simulink model "Hexa_CAD_quaternion_ANSFT"  (R2024b)
settings: Solver=ode4  StartTime=0.0  StopTime=60  FixedStep=0.01  RelTol=1e-3
model workspace (MAT data in the model file):
  hover_2m = [0 0 2 0 0 0 0 0 2 0 0 0 ... (36 elements, 6x6)]
  square = [0 0 2.5 0 0 0 0 0 2.5 0 0 0 ... (36 elements, 6x6)]
  tf : Simulink.Parameter (value not decoded)
  tray0 = [0 0 0 0 0 0 0.2 0.15 2 0 0 0 ... (36 elements, 6x6)]
  tray1 = [0 0 0 0 0 0 0 0 2 0 0 0 ... (36 elements, 6x6)]
  tray2 = [0 0 0 0 0 0 2 0 5 0 0 0 ... (36 elements, 6x6)]
  tray3 = [0 0 0 0 0 0 2 0 5 0 0 0 ... (36 elements, 6x6)]
  tray4 = [0 0 0 0 0 0 2 0 5 0.15 0 0 ... (36 elements, 6x6)]
  tray5 = [0 0 0 0 0 0 0 0 5 0.15 0 0 ... (36 elements, 6x6)]
  tray_yaw = [0 0 0 0 0 0 0 0 5 0 0 0 ... (36 elements, 6x6)]
undefined symbols (not defined in the file or in its folder): F, Light, MIL, smiData, X, Y, Z
libraries: sm_lib x167, nesl_utility x29, dspobslib x9, sharedtransform x4, simulink x4, aerolibutil x3, matrix_library x1, sharedutil x1, robotcorelib x1, aerolibwind2 x1
(part 3 of 6)

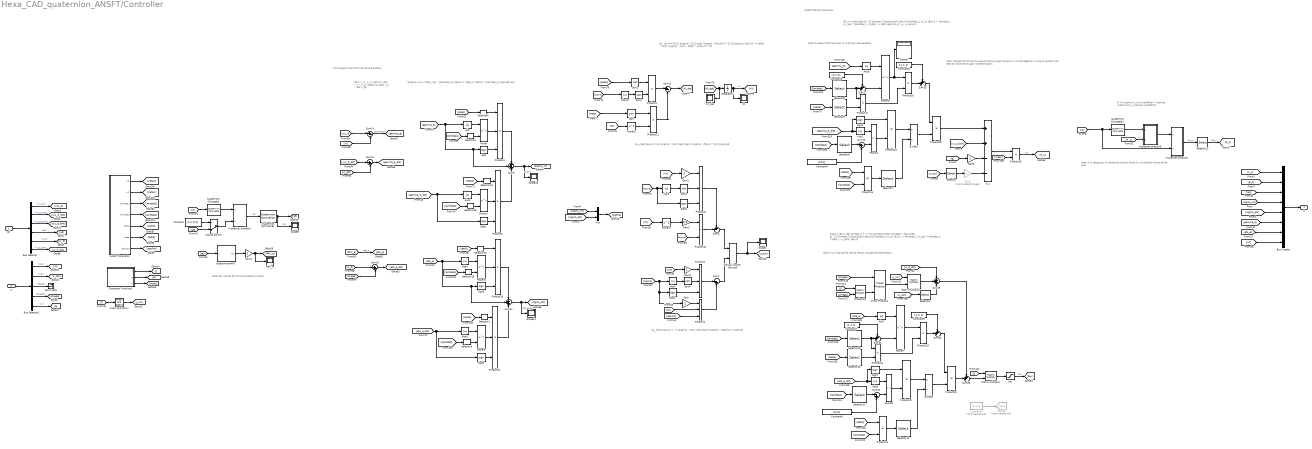
== system Hexa_CAD_quaternion_ANSFT/Controller ==
  note: $u_{\text{aux}}=-2K |\sigma|^{1/2} \text{sign} (\sigma) - \frac{K^2}{2}\sigma$
  note: $u_{\text{aux}} = - K |\sigma| ^{1/2} \text{sign}(\sigma) - 2\epsilon K \sigma$
  note: Note: PRV stands for Principal Rotation
      | Vector.
  note: $e = x_d - x_1 \\ \dot e = \dot x_d - x_2 \\ \ddot e = \ddot x_d - \dot x_2$
  note: Non-Singular Fast Terminal Sliding Surface
  note: $\sigma = e + \zeta_1 |e| ^{\lambda_1} sign(e) + \zeta_2 | \dot e| ^{\lambda_2} sign(\dot e)$
  note: $F_u = \frac{|\dot e|^{2-\lambda_2}\text{sign}(\dot e)}{\lambda_2 \xi_2} \Big (1 + \lambda_1 \xi_1|e|^{\lambda_1 - 1}\Big ) + \ddot \gamma_d - g - u_{aux}$
  note: Note: It seems that the mass is missing in
      | the equation.
  note: $\tau = \Big [ \dot \omega_d + J^{-1} \omega \times J \omega + \frac{|\dot e|^{2-\lambda_2}\text{sign}(\dot e)}{\lambda_2 \xi_2} \Big (1 + \lambda_1 \xi_1|e|^{\lambda_1 - 1}\Big ) - u_{aux} \Big ]$
  note: Note: Change the Thrust to a positive force, ergo the gravity will be negative,
      | will be using ENU over NED for future Simscape implementation.
  note: $^B \mathrm F_u = \mathbf{q}^*\otimes \mathrm{F}_u \otimes \mathbf q$
  note: ANSFT Position Controller
  note: Note: It is missing the Inertia Tensor outside
      | the parenthesis
  note: Note: It is necessary to rotate the control Force F_u
      | to the body frame of the FAH.
  note: $u_{aux}=-2K(t) |\sigma|^{1/2} sign (\sigma) - \frac{K(t)^2}{2}\sigma \\ \dot K(t) = \alpha ^{1/2} |\sigma| ^{1/2} - \beta ^{1/2}K(t)^2$
  qd : Inport
  q : Inport  Port=2
  ANSFT Constants : MATLAB Function  TreatAsAtomicUnit=on
  Abs{,1..10} (11 alike) : Abs  SaturateOnIntegerOverflow=off
  Bus Creator : BusCreator  Inputs=8
  Bus Selector : BusSelector  OutputSignals=xyz_d,xyz_d_dot,xyz_d_ddot,qd,w_d,w_d_dot
  Bus Selector1 : BusSelector  OutputSignals=pos,vel,bf_att,bf_datt,q
  Constant : Constant  Value=[1; 0; 0; 0]
  Constant{3,5,7,9} (4 alike) : Constant  Value=[1; 1; 1]
  Constant4 : Constant  Value=[2;2;2]
  Constant6 : Constant  Commented=on  Value=[0; 0; 0]
  Constant8 : Constant  Value=[2;2;2]
  Constants Functions : MATLAB Function  TreatAsAtomicUnit=on
  Cross Product1 : matrix_library/Cross Product
  Display : Display
  Divide2 : Product  Inputs=*/
  Divide3 : Product  Inputs=*/
  F_u : Sum  Inputs=++--
  Gain{,1,3..4} (4 alike) : Gain  Gain=2
  Gain2 : Gain  Gain=1/2
  Gain5 : Gain
  Gain6 : Gain  Commented=through  Gain=-1
  Goto59 : Goto  Commented=on  GotoTag=tau
  Integrator4 : Integrator  InitialCondition=[0;0;0; 0; 0; 0]
  Invert 3x3 Matrix : aerolibutil/Invert  3x3 Matrix
  Kronecker product4 : Subsystem
  Kronecker product6 : Subsystem
  Kronecker product7 : Subsystem
  Kt : Scope
  Kt_dot : Scope
  Manual Variant Source3 : simulink/Signal Routing/Manual Variant Source  NumChoices=2  LabelModeActiveChoice=V_2
  Manual Switch : ManualSwitch  CurrentSetting=0
  Matrix Multiply2 : Product  Multiplication=Matrix(*)
  Matrix Multiply5 : Product  Multiplication=Matrix(*)
  Mux : Mux  Inputs=2
  PRV_e : Scope
  Power{,1,4..9} (8 alike) : Math  Operator=pow
  Power2 : Math  Operator=square
  Power3 : Math  Operator=square
  Product{1..4,8,26..27} (7 alike) : Product  Inputs=3
  Product{9..11,13..18,20..24} (14 alike) : Product
  Product19 : Product  Multiplication=Matrix(*)
  Quaternion Conjugate : aerolibutil/Quaternion Conjugate
  Quaternion Conjugate1 : aerolibutil/Quaternion Conjugate
  Quaternion Normalize1 : sharedutil/Quaternion Normalize  aMode=aMode
  Scope{1,8,10,12} (4 alike) : Scope
  Selector{,4..9,15..16} (9 alike) : Selector  InputPortWidth=6  IndexOptions=Index vector (dialog)  Indices=[1:3]  OutputSizes=1
  Selector{1..3,10..14,18} (9 alike) : Selector  InputPortWidth=6  IndexOptions=Index vector (dialog)  Indices=[4:6]  OutputSizes=1
  Selector22 : Selector  InputPortWidth=4  IndexOptions=Index vector (dialog)  Indices=[2:4]  OutputSizes=1
  Sign{,1..7} (8 alike) : Signum
  Sqrt{,1..4} (5 alike) : Sqrt
  Sum1 : Sum  Inputs=|--
  Sum10 : Sum  Inputs=|-+
  Sum{11,14..16} (4 alike) : Sum  Inputs=|+-
  Sum17 : Sum  Inputs=-+|
  Sum18 : Sum  Inputs=++|
  Sum19 : Sum  Inputs=++-
  Sum20 : Sum  Inputs=|-+
  Sum21 : Sum  Inputs=-+|
  Sum22 : Sum  Inputs=++|
  Sum23 : Sum  Inputs=++|
  Sum24 : Sum  Inputs=+++
  Sum4 : Sum  Inputs=--|
  Sum9 : Sum  Inputs=+++
  Terminator : Terminator
  quaterniontoPRV : Subsystem
  tau : Saturate
  u : Outport
  wires:
  ANSFT Constants/4(lambda2) -> [lambda2]
  ANSFT Constants/6(beta) -> [beta]
  ANSFT Constants/3(lambda1) -> [lambda1]
  ANSFT Constants/1(xi1) -> [zeta1]
  ANSFT Constants/5(alpha) -> [alpha]
  ANSFT Constants/2(xi2) -> [zeta2]
  qd/1 -> Bus Selector/1
  Constants Functions/1(J) -> [J]
  Bus Creator/1 -> u/1
  q/1 -> Bus Selector1/1
  Bus Selector1/1 -> [xi]  "<pos>"
  Bus Selector1/3 -> Terminator/1  "<bf_att>"
  Bus Selector1/2 -> [xi_dot]  "<vel>"
  Bus Selector1/4 -> [omega]  "<bf_datt>"
  ANSFT Constants/7(epsilon) -> [epsilon]
  Abs4/1 -> Sqrt4/1
  Gain3/1 -> Product1/1
  Sum4/1 -> Manual Variant Source3/1
  Manual Variant Source3/1 -> Scope1/1, [u_aux]
  Sign4/1 -> Product1/3
  Product8/1 -> Sum4/1
  Product10/1 -> Sum4/2
  Power3/1 -> Gain2/1
  [epsilon] -> Product2/3
  Gain1/1 -> Product8/1
  Gain/1 -> Product2/1
  [Kt] -> Gain1/1
  Product1/1 -> Sum1/1
  Sum1/1 -> Manual Variant Source3/2
  [sigma] -> Product10/2
  Gain2/1 -> Product10/1
  [sigma] -> Abs4/1, Gain/1, Sign4/1
  Sqrt3/1 -> Product8/2
  Product2/1 -> Sum1/2
  Sqrt4/1 -> Product1/2
  [Kt] -> Gain3/1
  [Kt] -> Product2/2
  Abs3/1 -> Sqrt3/1
  [sigma] -> Sign3/1, Abs3/1
  [Kt] -> Power3/1
  Sign3/1 -> Product8/3
  Bus Selector/1 -> [xyz_d]  "<xyz_d>"
  Bus Selector/4 -> [qd]  "<qd>"
  Bus Selector/5 -> [w_d]  "<w_d>"
  Bus Selector/6 -> [w_d_dot]  "<w_d_dot>"
  Bus Selector/2 -> [xyz_d_dot]  "<xyz_d_dot>"
  Bus Selector/3 -> [xyz_d_ddot]  "<xyz_d_ddot>"
  Bus Selector1/5 -> [q]  "<q>"
  Invert 3x3 Matrix/1 -> [J_inv]
  [J] -> Invert 3x3 Matrix/1
  Kronecker product4/1(r) -> Quaternion Normalize1/1  "qe"
  Constant/1 -> Manual Switch/1
  Gain4/1 -> PRV_e/1, [PRV_e]
  [q] -> Quaternion Conjugate/1
  Quaternion Conjugate/1 -> Kronecker product4/1(q)
  [qe] -> quaterniontoPRV/1(q)
  Quaternion Normalize1/1 -> Scope8/1, [qe]  "qe"
  [qd] -> Manual Switch/2
  quaterniontoPRV/1(lnq) -> Gain4/1
  Manual Switch/1 -> Kronecker product4/2(p)
  [eta_e] -> Sum24/2, Sign5/1, Abs8/1
  Selector18/1 -> Power8/2
  Sum24/1 -> Scope10/1, [sigma_att]  "sigma_att"
  Sum15/1 -> [gamma_e_dot]
  [xyz_d] -> Sum14/1
  Sign/1 -> Product4/3
  Selector4/1 -> Product4/1
  Power/1 -> Product4/2
  Selector3/1 -> Power9/2
  [xyz_d_dot] -> Sum15/1
  Product27/1 -> Sum24/3
  [PRV_e] -> [eta_e]  "eta_e"
  [zeta2] -> Selector1/1
  [lambda2] -> Selector16/1
  Abs8/1 -> Power8/1
  [eta_e_dot] -> Abs9/1, Sign6/1
  Selector16/1 -> Power1/2
  Product26/1 -> Sum24/1
  [lambda2] -> Selector3/1
  [gamma_e_dot] -> Sign1/1, Abs1/1
  [xi] -> Sum14/2
  Sign5/1 -> Product26/3
  [gamma_e] -> Sum9/2, Sign/1, Abs/1
  Sign1/1 -> Product3/3
  [xi_dot] -> Sum15/2
  Sum9/1 -> Scope12/1, [sigma_lin]  "sigma"
  [omega] -> Sum16/2
  [zeta2] -> Selector15/1
  [lambda1] -> Selector5/1
  [w_d] -> Sum16/1
  Selector5/1 -> Power/2
  Power9/1 -> Product27/2
  [zeta1] -> Selector10/1
  Abs9/1 -> Power9/1
  [zeta1] -> Selector4/1
  Abs/1 -> Power/1
  Sum14/1 -> [gamma_e]  "gamma_e"
  [lambda1] -> Selector18/1
  Power1/1 -> Product3/2
  Selector10/1 -> Product26/1
  Product4/1 -> Sum9/1
  Selector1/1 -> Product27/1
  Sum16/1 -> [eta_e_dot]
  Sign6/1 -> Product27/3
  Product3/1 -> Sum9/3
  Abs1/1 -> Power1/1
  Selector15/1 -> Product3/1
  Power8/1 -> Product26/2
  [sigma_lin] -> Mux/1
  [sigma_att] -> Mux/2
  Mux/1 -> [sigma]
  Sum20/1 -> Power6/2
  Product13/1 -> Divide2/1
  [g] -> Gain5/1
  Product20/1 -> Divide3/1
  Sum21/1 -> Power7/2
  [J_inv] -> Matrix Multiply2/1
  Constant9/1 -> Sum22/1
  Selector8/1 -> Product17/1, Sum17/2
  [J] -> Product19/1
  [w_d_dot] -> Sum19/1
  Abs2/1 -> Power4/1
  Cross Product1/1 -> Matrix Multiply2/2
  [eta_e_dot] -> Sign7/1, Abs6/1
  [zeta2] -> Product14/1
  Constant3/1 -> Sum17/1
  [eta_e] -> Abs7/1
  Abs7/1 -> Power7/1
  Selector7/1 -> Divide2/2
  [zeta1] -> Selector14/1
  Constant8/1 -> Sum20/2
  Product23/1 -> Sum22/2
  Matrix Multiply5/1 -> tau/1
  Selector14/1 -> Product24/2
  Selector9/1 -> Product17/2
  Sum10/1 -> Power4/2
  Abs5/1 -> Power5/1
  [zeta2] -> Product21/1
  Kronecker product6/1(r) -> Kronecker product7/1(q)
  [lambda2] -> Product14/2
  [lambda1] -> Selector8/1
  Gain5/1 -> F_u/3
  [J] -> Matrix Multiply5/1
  Sum18/1 -> Product15/1
  [zeta1] -> Selector9/1
  Selector12/1 -> Divide3/2
  Selector13/1 -> Product24/1, Sum21/2
  [omega] -> Product19/2
  Power5/1 -> Display/1, Product16/1
  Product15/1 -> F_u/1
  Constant7/1 -> Sum21/1
  Selector6/1 -> Sum10/1
  [u_aux] -> Selector/1
  Product24/1 -> Product23/2
  Sign7/1 -> Product20/1
  [xyz_d_ddot] -> F_u/2
  Sign2/1 -> Product13/1
  Product21/1 -> Selector12/1
  [lambda2] -> Selector6/1
  [lambda2] -> Product21/2
  F_u/1 -> Product18/1
  Product22/1 -> Sum23/2
  [mass] -> Product18/2
  Product14/1 -> Selector7/1
  Abs6/1 -> Power6/1
  Product16/1 -> Sum18/2
  [gamma_e_dot] -> Sign2/1, Abs2/1
  Product18/1 -> [F_u]  "F_u"
  Selector22/1 -> [B_F]  "B-F_u"
  Constant4/1 -> Sum10/2
  Power4/1 -> Product13/2
  [omega] -> Cross Product1/1
  Product19/1 -> Cross Product1/2
  [lambda2] -> Selector11/1
  Divide3/1 -> Product22/2
  Matrix Multiply2/1 -> Sum19/2
  Gain6/1 -> F_u/4
  Selector11/1 -> Sum20/1
  Divide2/1 -> Product15/2
  Sum19/1 -> Sum23/1
  [gamma_e] -> Abs5/1
  Product17/1 -> Product16/2
  Sum22/1 -> Product22/1
  Sum23/1 -> Matrix Multiply5/2
  Constant5/1 -> Sum18/1
  [F_u] -> Kronecker product6/2(p)  "fu"
  [lambda1] -> Selector13/1
  Constant6/1 -> Goto59/1
  [u_aux] -> Selector2/1
  tau/1 -> [tau]  "tau"
  [q] -> Kronecker product7/2(p), Quaternion Conjugate1/1
  Quaternion Conjugate1/1 -> Kronecker product6/1(q)
  Kronecker product7/1(r) -> Selector22/1  "B_F_u"
  Sum17/1 -> Power5/2
  Power6/1 -> Product20/2
  Power7/1 -> Product23/1
  [B_F] -> Bus Creator/2
  [Kt] -> Bus Creator/8
  [eta_e] -> Bus Creator/7
  [sigma_lin] -> Bus Creator/4
  [gamma_e] -> Bus Creator/6
  [tau] -> Bus Creator/3
  [sigma_att] -> Bus Creator/5
  [F_u] -> Bus Creator/1
  Integrator4/1 -> Kt/1, [Kt]  "Kt"
  Product9/1 -> Sum11/1
  [Kt_dot] -> Kt_dot/1, Integrator4/1
  [beta] -> Sqrt/1
  [sigma] -> Abs10/1
  [alpha] -> Sqrt1/1
  Sqrt1/1 -> Product9/1
  Product11/1 -> Sum11/2
  Abs10/1 -> Sqrt2/1
  Sqrt2/1 -> Product9/2
  [Kt] -> Power2/1
  Sum11/1 -> [Kt_dot]
  Sqrt/1 -> Product11/1
  Power2/1 -> Product11/2
  Constants Functions/2(g) -> [g]
  Constants Functions/3(m) -> [mass]
  Selector/1 -> Gain6/1
  Selector2/1 -> Sum19/3

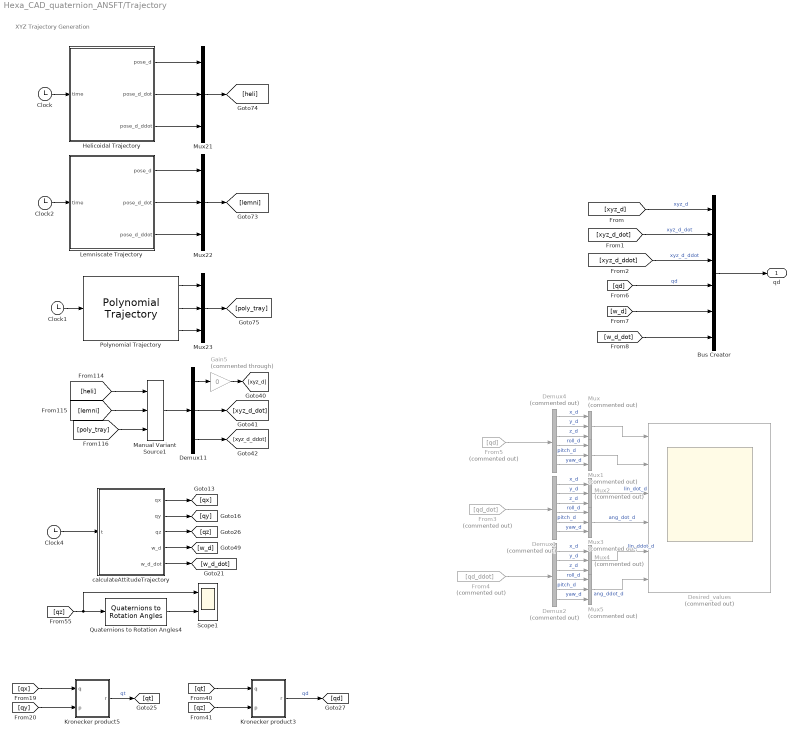
== system Hexa_CAD_quaternion_ANSFT/Trajectory ==
  note: XYZ Trajectory Generation
  Bus Creator : BusCreator  Inputs=6
  Clock{,1..2,4} (4 alike) : Clock
  Demux1 : Demux  Commented=on  Outputs=6
  Demux11 : Demux  Outputs=3
  Demux2 : Demux  Commented=on  Outputs=6
  Demux4 : Demux  Commented=on  Outputs=6
  Desired_values : Scope  Commented=on  NumInputPorts=6
  From3 : From  Commented=on  GotoTag=qd_dot
  From4 : From  Commented=on  GotoTag=qd_ddot
  From5 : From  Commented=on  GotoTag=qd
  Gain5 : Gain  Commented=through  Gain=0
  Helicoidal Trajectory : MATLAB Function  TreatAsAtomicUnit=on
  Kronecker product3 : Subsystem
  Kronecker product5 : Subsystem
  Lemniscate Trajectory : MATLAB Function  TreatAsAtomicUnit=on
  Manual Variant Source1 : simulink/Signal Routing/Manual Variant Source  NumChoices=3  LabelModeActiveChoice=V_1
  Mux{,1..5} (6 alike) : Mux  Commented=on  Inputs=3
  Mux21 : Mux  Inputs=3
  Mux22 : Mux  Inputs=3
  Mux23 : Mux  Inputs=3
  Polynomial Trajectory : robotcorelib/Polynomial Trajectory  WaypointSource=Internal  Waypoints=zeros(3, 6)  TimePoints=[ 0, 12, 24, 36, 48, 60]  TimeInterval=[ 1, 4 ]  Method=Cubic Polynomial  ParameterSource=Internal  VelocityBoundaryCondition=zeros( 3, 6)  AccelerationBoundaryCondition=zeros( 2, 5 )  SimulateUsing=Interpreted execution
  Quaternions to Rotation Angles4 : sharedtransform/Quaternions to Rotation Angles  rotationOrder=ZYX  aMode=aMode
  Scope1 : Scope  NumInputPorts=2
  calculateAttitudeTrajectory : MATLAB Function  TreatAsAtomicUnit=on
  qd : Outport
  wires:
  Demux4/1 -> Mux/1  "x_d"
  Demux2/5 -> Mux5/2  "pitch_d"
  Demux1/5 -> Mux3/2  "pitch_d"
  Demux1/3 -> Mux2/3  "z_d"
  Demux4/6 -> Mux1/3  "yaw_d"
  From3/1 -> Demux1/1
  Demux1/2 -> Mux2/2  "y_d"
  Mux1/1 -> Desired_values/2
  Demux4/3 -> Mux/3  "z_d"
  Demux4/2 -> Mux/2  "y_d"
  Demux1/1 -> Mux2/1  "x_d"
  From4/1 -> Demux2/1
  Mux2/1 -> Desired_values/3  "lin_dot_d"
  Demux4/5 -> Mux1/2  "pitch_d"
  Mux5/1 -> Desired_values/6  "ang_ddot_d"
  Demux2/3 -> Mux4/3  "z_d"
  From5/1 -> Demux4/1
  Mux3/1 -> Desired_values/4  "ang_dot_d"
  Demux4/4 -> Mux1/1  "roll_d"
  Mux/1 -> Desired_values/1
  Demux1/4 -> Mux3/1  "roll_d"
  Demux2/1 -> Mux4/1  "x_d"
  Demux1/6 -> Mux3/3  "yaw_d"
  Mux4/1 -> Desired_values/5  "lin_ddot_d"
  Bus Creator/1 -> qd/1
  Demux2/4 -> Mux5/1  "roll_d"
  Demux2/6 -> Mux5/3  "yaw_d"
  Demux2/2 -> Mux4/2  "y_d"
  [lemni] -> Manual Variant Source1/2
  Clock1/1 -> Polynomial Trajectory/1
  Gain5/1 -> [xyz_d]
  calculateAttitudeTrajectory/3(qz) -> [qz]
  Helicoidal Trajectory/1(pose_d) -> Mux21/1
  [poly_tray] -> Manual Variant Source1/3
  [qz] -> Scope1/1, Quaternions to Rotation Angles4/1
  Polynomial Trajectory/3 -> Mux23/3
  Helicoidal Trajectory/2(pose_d_dot) -> Mux21/2
  Demux11/1 -> Gain5/1
  Demux11/3 -> [xyz_d_ddot]
  Clock4/1 -> calculateAttitudeTrajectory/1(t)
  Lemniscate Trajectory/2(pose_d_dot) -> Mux22/2
  calculateAttitudeTrajectory/1(qx) -> [qx]
  calculateAttitudeTrajectory/2(qy) -> [qy]
  calculateAttitudeTrajectory/5(w_d_dot) -> [w_d_dot]
  Clock/1 -> Helicoidal Trajectory/1(time)
  [heli] -> Manual Variant Source1/1
  calculateAttitudeTrajectory/4(w_d) -> [w_d]
  Polynomial Trajectory/1 -> Mux23/1
  Clock2/1 -> Lemniscate Trajectory/1(time)
  Demux11/2 -> [xyz_d_dot]
  Mux22/1 -> [lemni]
  Helicoidal Trajectory/3(pose_d_ddot) -> Mux21/3
  Lemniscate Trajectory/3(pose_d_ddot) -> Mux22/3
  Lemniscate Trajectory/1(pose_d) -> Mux22/1
  Mux23/1 -> [poly_tray]
  Manual Variant Source1/1 -> Demux11/1
  Quaternions to Rotation Angles4/1 -> Scope1/2
  Polynomial Trajectory/2 -> Mux23/2
  Mux21/1 -> [heli]
  [w_d_dot] -> Bus Creator/6
  [qd] -> Bus Creator/4  "qd"
  [w_d] -> Bus Creator/5
  [xyz_d_ddot] -> Bus Creator/3  "xyz_d_ddot"
  [xyz_d_dot] -> Bus Creator/2  "xyz_d_dot"
  [xyz_d] -> Bus Creator/1  "xyz_d"
  [qx] -> Kronecker product5/1(q)
  Kronecker product3/1(r) -> [qd]  "qd"
  [qz] -> Kronecker product3/2(p)
  [qt] -> Kronecker product3/1(q)
  Kronecker product5/1(r) -> [qt]  "qt"
  [qy] -> Kronecker product5/2(p)

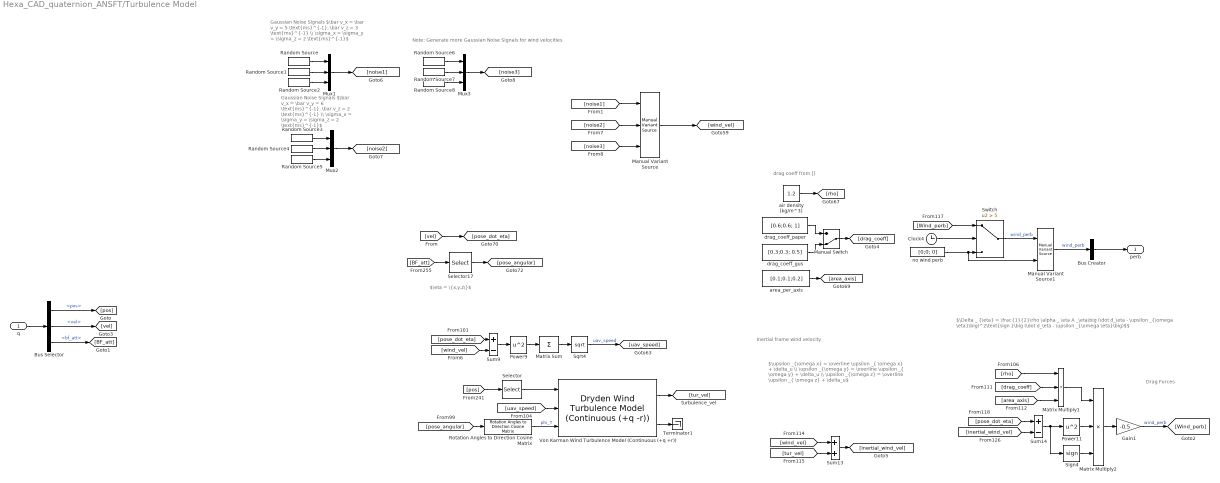
== system Hexa_CAD_quaternion_ANSFT/Turbulence Model ==
  note: Note: Generate more Gaussian Noise Signals
      | for wind velocities
  note: $\Delta _ {\eta} = \frac{1}{2}\rho \alpha _ \eta A _\eta\big (\dot d_\eta - \upsilon _{\omega \eta}\big)^2\text{sign }\big (\dot d_\eta - \upsilon _{\omega \eta}\big)$$
  note: $\upsilon _{\omega x} = \overline \upsilon _{ \omega x} + \delta_u \\ \upsilon _{\omega y} = \overline \upsilon _{ \omega y} + \delta_u \\ \upsilon _{\omega z} = \overline \upsilon _{ \omega z} + \delta_u$
  note: drag coeff from []
  note: Drag Forces
  note: Inertial frame wind velocity
  note: $\eta = \{x,y,z\}$
  note: Gaussian Noise Signals
      | $\bar v_x = \bar v_y = 6 \text{ms}^{-1}, \bar v_z = 2 \text{ms}^{-1} \\ \sigma_x = \sigma_y = \sigma_z = 2 \text{ms}^{-1}$
  note: Gaussian Noise Signals
      | $\bar v_x = \bar v_y = 5 \text{ms}^{-1}, \bar v_z = 3 \text{ms}^{-1} \\ \sigma_x = \sigma_y = \sigma_z = 2 \text{ms}^{-1}$
  q : Inport
  Bus Creator : BusCreator  Inputs=1
  Bus Selector : BusSelector  OutputSignals=pos,vel,bf_att
  Clock4 : Clock
  Gain1 : Gain  Gain=-0.5
  Manual Variant Source : simulink/Signal Routing/Manual Variant Source  NumChoices=3  LabelModeActiveChoice=V_1
  Manual Variant Source1 : simulink/Signal Routing/Manual Variant Source  NumChoices=2  LabelModeActiveChoice=V_1
  Manual Switch : ManualSwitch  CurrentSetting=0
  Matrix Sum : Sum  Inputs=+
  Matrix Multiply1 : Product  Inputs=3
  Matrix Multiply2 : Product  Inputs=3
  Mux1 : Mux  Inputs=3
  Mux2 : Mux  Inputs=3
  Mux3 : Mux  Inputs=3
  Power11 : Math  Operator=square
  Power9 : Math  Operator=square
  Random Source : dspobslib/Random Source  SrcType=Gaussian  NormMethod=Ziggurat  CltLength=12  MinVal=0  MaxVal=1  MeanVal=5  VarVal=2  RepMode=Not repeatable  rawSeed=1  IsInherit=off  SampMode=Discrete  SampTime=1  SampFrame=1  DataType=Double  OutComplex=Real  OutputFrames=off
  Random Source1 : dspobslib/Random Source  SrcType=Gaussian  NormMethod=Ziggurat  CltLength=12  MinVal=0  MaxVal=1  MeanVal=5  VarVal=2  RepMode=Not repeatable  rawSeed=1  IsInherit=off  SampMode=Discrete  SampTime=1  SampFrame=1  DataType=Double  OutComplex=Real  OutputFrames=off
  Random Source2 : dspobslib/Random Source  SrcType=Gaussian  NormMethod=Ziggurat  CltLength=12  MinVal=0  MaxVal=1  MeanVal=3  VarVal=2  RepMode=Not repeatable  rawSeed=1  IsInherit=off  SampMode=Discrete  SampTime=1  SampFrame=1  DataType=Double  OutComplex=Real  OutputFrames=off
  Random Source{3..4,6..7} (4 alike) : dspobslib/Random Source  SrcType=Gaussian  NormMethod=Ziggurat  CltLength=12  MinVal=0  MaxVal=1  MeanVal=6  VarVal=2  RepMode=Not repeatable  rawSeed=1  IsInherit=off  SampMode=Discrete  SampTime=1  SampFrame=1  DataType=Double  OutComplex=Real  OutputFrames=off
  Random Source5 : dspobslib/Random Source  SrcType=Gaussian  NormMethod=Ziggurat  CltLength=12  MinVal=0  MaxVal=1  MeanVal=2  VarVal=2  RepMode=Not repeatable  rawSeed=1  IsInherit=off  SampMode=Discrete  SampTime=1  SampFrame=1  DataType=Double  OutComplex=Real  OutputFrames=off
  Random Source8 : dspobslib/Random Source  SrcType=Gaussian  NormMethod=Ziggurat  CltLength=12  MinVal=0  MaxVal=1  MeanVal=2  VarVal=2  RepMode=Not repeatable  rawSeed=1  IsInherit=off  SampMode=Discrete  SampTime=1  SampFrame=1  DataType=Double  OutComplex=Real  OutputFrames=off
  Rotation Angles to Direction Cosine Matrix : sharedtransform/Rotation Angles to Direction Cosine Matrix  rotationOrder=XYZ  aMode=aMode
  Selector : Selector  InputPortWidth=3  IndexOptions=Index vector (dialog)  Indices=[3]  OutputSizes=1
  Selector17 : Selector  InputPortWidth=3  IndexOptions=Index vector (dialog)  Indices=[3 2 1]  OutputSizes=1
  Sign4 : Signum
  Sqrt4 : Sqrt
  Sum13 : Sum
  Sum14 : Sum  Inputs=+-
  Sum9 : Sum  Inputs=+-
  Switch : Switch  Criteria=u2 > Threshold  Threshold=5  SaturateOnIntegerOverflow=off  InputSameDT=off
  Terminator1 : Terminator
  Von Karman Wind Turbulence Model (Continuous (+q +r)) : aerolibwind2/Dryden Wind Turbulence Model  (Continuous (+q -r))  units=Metric (MKS)  spec=MIL-F-8785C  model=Continuous Von Karman (+q -r)  W20=15  Wdeg=0  TurbProb=10^-2 - Light  L_high=762  Wingspan=10  ts=0.1  Seed=[23341 23342 23343 23344]  T_on=on
      settings: LibrarySourceBlock=|
      | aerolibwind2/Von Karman Wind Turbulence Model
      | (Continuous (+q +r))
  air density [kg/m^3] : Constant  Value=1.2
  area_per_axis : Constant  Value=[0.1;0.1;0.2]
  drag_coeff_gus : Constant  Value=[0.3;0.3; 0.5]
  drag_coeff_paper : Constant  Value=[0.6;0.6; 1]
  no wind perb : Constant  Value=[0;0; 0]
  perb : Outport
  wires:
  [rho] -> Matrix Multiply1/1
  [drag_coeff] -> Matrix Multiply1/2
  Von Karman Wind Turbulence Model (Continuous (+q +r))/2 -> Terminator1/1
  area_per_axis/1 -> [area_axis]
  [pose_dot_eta] -> Sum14/1
  Von Karman Wind Turbulence Model (Continuous (+q +r))/1 -> [tur_vel]
  [wind_vel] -> Sum9/2
  Selector17/1 -> [pose_angular]
  Matrix Multiply1/1 -> Matrix Multiply2/1
  Sign4/1 -> Matrix Multiply2/3
  [uav_speed] -> Von Karman Wind Turbulence Model (Continuous (+q +r))/2
  Power9/1 -> Matrix Sum/1
  Sqrt4/1 -> [uav_speed]  "uav_speed"
  Gain1/1 -> [Wind_perb]  "wind_perb"
  Sum9/1 -> Power9/1
  air density [kg/m^3]/1 -> [rho]
  Clock4/1 -> Switch/2
  [pose_dot_eta] -> Sum9/1
  Rotation Angles to Direction Cosine Matrix/1 -> Von Karman Wind Turbulence Model (Continuous (+q +r))/3  "phi_T"
  [tur_vel] -> Sum13/2
  Sum14/1 -> Sign4/1, Power11/1
  no wind perb/1 -> Manual Variant Source1/2, Switch/3
  drag_coeff_gus/1 -> Manual Switch/2
  Switch/1 -> Manual Variant Source1/1  "wind_perb"
  [area_axis] -> Matrix Multiply1/3
  Manual Switch/1 -> [drag_coeff]
  Selector/1 -> Von Karman Wind Turbulence Model (Continuous (+q +r))/1
  [pose_angular] -> Rotation Angles to Direction Cosine Matrix/1
  [inertial_wind_vel] -> Sum14/2
  Matrix Multiply2/1 -> Gain1/1
  drag_coeff_paper/1 -> Manual Switch/1
  Power11/1 -> Matrix Multiply2/2
  Matrix Sum/1 -> Sqrt4/1
  Sum13/1 -> [inertial_wind_vel]
  [Wind_perb] -> Switch/1
  [wind_vel] -> Sum13/1
  Bus Creator/1 -> perb/1
  [BF_att] -> Selector17/1
  [pos] -> Selector/1
  q/1 -> Bus Selector/1
  Bus Selector/1 -> [pos]  "<pos>"
  Bus Selector/3 -> [BF_att]  "<bf_att>"
  Bus Selector/2 -> [vel]  "<vel>"
  [vel] -> [pose_dot_eta]
  Mux2/1 -> [noise2]
  Random Source5/1 -> Mux2/3
  Random Source/1 -> Mux1/1
  Mux1/1 -> [noise1]
  Random Source2/1 -> Mux1/3
  Random Source4/1 -> Mux2/2
  Random Source3/1 -> Mux2/1
  [noise2] -> Manual Variant Source/2
  Manual Variant Source/1 -> [wind_vel]
  Random Source1/1 -> Mux1/2
  [noise1] -> Manual Variant Source/1
  [noise3] -> Manual Variant Source/3
  Mux3/1 -> [noise3]
  Random Source7/1 -> Mux3/2
  Random Source6/1 -> Mux3/1
  Random Source8/1 -> Mux3/3
  Manual Variant Source1/1 -> Bus Creator/1  "wind_perb"

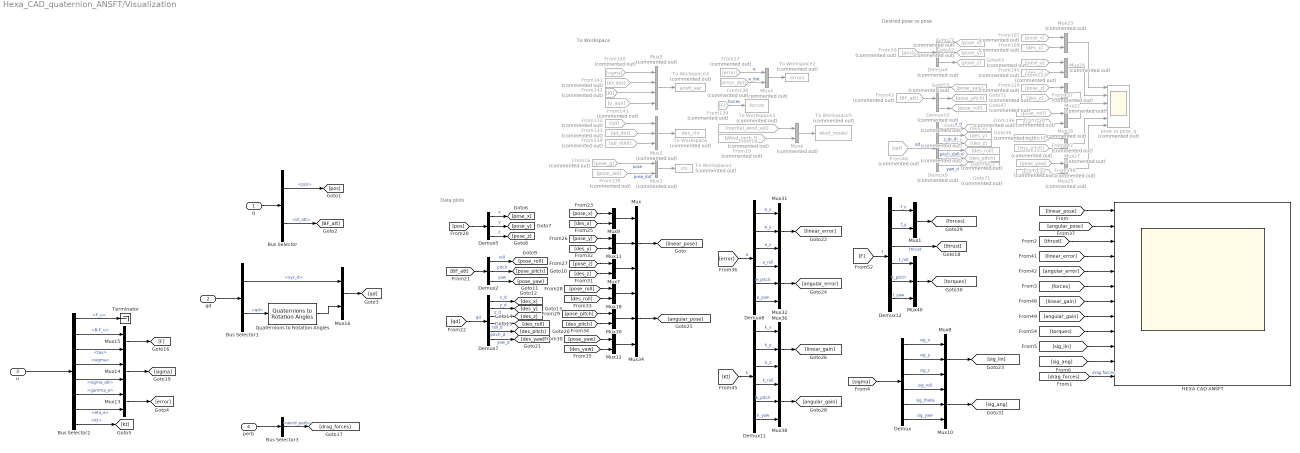
== system Hexa_CAD_quaternion_ANSFT/Visualization ==
  note: Desired pose vs pose
  note: Data plots
  note: To Workspace
  q : Inport
  qd : Inport  Port=2
  u : Inport  Port=3
  perb : Inport  Port=4
  Bus Selector : BusSelector  OutputSignals=pos,bf_att
  Bus Selector1 : BusSelector  OutputSignals=xyz_d,qd
  Bus Selector2 : BusSelector  OutputSignals=F_u,B-F_u,tau,sigma,sigma_att,gamma_e,eta_e,Kt
  Bus Selector3 : BusSelector  OutputSignals=wind_perb
  Demux{,7..8,11..12} (5 alike) : Demux  Outputs=6
  Demux10 : Demux  Commented=on  Outputs=3
  Demux2 : Demux  Outputs=3
  Demux4 : Demux  Commented=on  Outputs=3
  Demux5 : Demux  Outputs=3
  Demux9 : Demux  Commented=on  Outputs=6
  From107 : From  Commented=on  GotoTag=pose_x
  From109 : From  Commented=on  GotoTag=des_x
  From122 : From  Commented=on  GotoTag=pose_y
  From124 : From  Commented=on  GotoTag=pose_z
  From128 : From  Commented=on  GotoTag=pose_roll
  From131 : From  Commented=on  GotoTag=pose_pitch
  From132 : From  Commented=on  GotoTag=qd
  From133 : From  Commented=on  GotoTag=qd_dot
  From134 : From  Commented=on  GotoTag=qd_ddot
  From135 : From  Commented=on  GotoTag=pose_yaw
  From136 : From  Commented=on  GotoTag=pose_dot
  From137 : From  Commented=on  GotoTag=des_z
  From138 : From  Commented=on  GotoTag=error_dot
  From139 : From  Commented=on  GotoTag=F
  From140 : From  Commented=on  GotoTag=sigma
  From141 : From  Commented=on  GotoTag=Kt_dot
  From142 : From  Commented=on  GotoTag=Kt
  From143 : From  Commented=on  GotoTag=u_aux
  From145 : From  Commented=on  GotoTag=des_y
  From146 : From  Commented=on  GotoTag=des_roll
  From147 : From  Commented=on  GotoTag=des_pitch
  From148 : From  Commented=on  GotoTag=des_yaw
  From16 : From  Commented=on  GotoTag=pose_g
  From17 : From  Commented=on  GotoTag=error
  From18 : From  Commented=on  GotoTag=inertial_wind_vel
  From19 : From  Commented=on  GotoTag=Wind_perb_f  TagVisibility=global
  From39 : From  Commented=on  GotoTag=pos
  From43 : From  Commented=on  GotoTag=BF_att
  From44 : From  Commented=on  GotoTag=qd
  Goto27 : Goto  Commented=on  GotoTag=pose_x
  Goto42 : Goto  Commented=on  GotoTag=pose_y
  Goto43 : Goto  Commented=on  GotoTag=pose_z
  Goto47 : Goto  Commented=on  GotoTag=pose_roll
  Goto51 : Goto  Commented=on  GotoTag=pose_pitch
  Goto53 : Goto  Commented=on  GotoTag=pose_yaw
  Goto55 : Goto  Commented=on  GotoTag=des_x
  Goto56 : Goto  Commented=on  GotoTag=des_y
  Goto57 : Goto  Commented=on  GotoTag=des_z
  Goto60 : Goto  Commented=on  GotoTag=des_roll
  Goto68 : Goto  Commented=on  GotoTag=des_pitch
  Goto71 : Goto  Commented=on  GotoTag=des_yaw
  HEXA CAD ANSFT : Scope  NumInputPorts=12
  Mux{,8,10,31..32,34,36,38,40} (9 alike) : Mux  Inputs=3
  Mux{1,7,9,11..16,18,30} (11 alike) : Mux  Inputs=2
  Mux2 : Mux  Commented=on  Inputs=3
  Mux{3..4,6,22..27} (9 alike) : Mux  Commented=on  Inputs=2
  Mux5 : Mux  Commented=on
  Quaternions to Rotation Angles : sharedtransform/Quaternions to Rotation Angles  rotationOrder=XYZ  aMode=aMode
  Terminator : Terminator
  To Workspace : ToWorkspace  Commented=on  VariableName=des_chi  SaveFormat=Structure With Time  SampleTime=-1
  To Workspace1 : ToWorkspace  Commented=on  VariableName=chi  SaveFormat=Structure With Time  SampleTime=-1
  To Workspace2 : ToWorkspace  Commented=on  VariableName=errors  SaveFormat=Structure With Time  SampleTime=-1
  To Workspace3 : ToWorkspace  Commented=on  VariableName=forces  SaveFormat=Structure With Time  SampleTime=-1
  To Workspace4 : ToWorkspace  Commented=on  VariableName=ansft_var  SaveFormat=Structure With Time  SampleTime=-1
  To Workspace5 : ToWorkspace  Commented=on  VariableName=wind_model  SaveFormat=Structure With Time  SampleTime=-1
  pose vs pose_q : Scope  Commented=on  NumInputPorts=6
  wires:
  Mux/1 -> [linear_pose]
  Mux6/1 -> To Workspace5/1
  Mux9/1 -> Mux/1
  From128/1 -> Mux26/1
  Demux4/1 -> Goto27/1
  Demux7/5 -> [des_pitch]  "pitch_d"
  From135/1 -> Mux25/1
  [linear_error] -> HEXA CAD ANSFT/4
  [angular_error] -> HEXA CAD ANSFT/5
  From132/1 -> Mux2/1
  Mux11/1 -> Mux/2
  Demux11/2 -> Mux36/2  "k_y"
  Demux4/3 -> Goto43/1
  Demux5/1 -> [pose_x]  "x"
  Demux10/1 -> Goto53/1
  Demux12/6 -> Mux40/3  "t_yaw"
  Demux12/4 -> Mux40/1  "t_roll"
  Mux40/1 -> [torques]
  Mux1/1 -> [forces]
  Demux10/3 -> Goto47/1
  Mux3/1 -> To Workspace1/1
  Demux5/3 -> [pose_z]  "z"
  Demux11/1 -> Mux36/1  "k_x"
  Demux8/6 -> Mux32/3  "e_yaw"
  From148/1 -> Mux25/2
  Demux11/4 -> Mux38/1  "k_roll"
  Demux9/6 -> Goto71/1  "yaw_d"
  [BF_att] -> Demux2/1
  Mux31/1 -> [linear_error]
  Mux23/1 -> pose vs pose_q/1
  Demux9/2 -> Goto56/1  "y_d"
  Demux7/2 -> [des_y]  "y_d"
  Demux5/2 -> [pose_y]  "y"
  From16/1 -> Mux3/1  "pose"
  [pose_pitch] -> Mux30/1
  [pose_y] -> Mux11/1
  Demux8/3 -> Mux31/3  "e_z"
  From44/1 -> Demux9/1  "qd"
  Demux7/3 -> [des_z]  "z_d"
  Demux12/2 -> Mux1/2  "f_y"
  [angular_gain] -> HEXA CAD ANSFT/8
  [error] -> Demux8/1  "e"
  From133/1 -> Mux2/2
  [des_pitch] -> Mux30/2
  [F] -> Demux12/1  "f"
  Mux5/1 -> To Workspace4/1
  [linear_gain] -> HEXA CAD ANSFT/7
  Mux2/1 -> To Workspace/1
  [des_roll] -> Mux18/2
  From43/1 -> Demux10/1
  Mux22/1 -> pose vs pose_q/3
  Mux26/1 -> pose vs pose_q/4
  Mux24/1 -> pose vs pose_q/2
  Demux12/1 -> Mux1/1  "f_x"
  From109/1 -> Mux23/2
  Demux7/4 -> [des_roll]  "roll_d"
  Demux9/4 -> Goto60/1  "roll_d"
  Demux12/3 -> [thrust]  "thrust"
  From122/1 -> Mux24/1
  Mux36/1 -> [linear_gain]
  [des_yaw] -> Mux12/2
  Demux11/6 -> Mux38/3  "k_yaw"
  From139/1 -> To Workspace3/1  "forces"
  [angular_pose] -> HEXA CAD ANSFT/2
  Demux9/3 -> Goto57/1  "z_d"
  Demux8/1 -> Mux31/1  "e_x"
  From124/1 -> Mux22/1
  Demux7/1 -> [des_x]  "x_d"
  From138/1 -> Mux4/2  "e_dot"
  [pose_yaw] -> Mux12/1
  From39/1 -> Demux4/1
  From137/1 -> Mux22/2
  Mux12/1 -> Mux34/3
  From131/1 -> Mux27/1
  Demux12/5 -> Mux40/2  "t_pitch"
  [des_x] -> Mux9/2
  Demux8/4 -> Mux32/1  "e_roll"
  [linear_pose] -> HEXA CAD ANSFT/1
  Demux9/1 -> Goto55/1  "x_d"
  [pos] -> Demux5/1
  From18/1 -> Mux6/1
  From141/1 -> Mux5/2
  Mux7/1 -> Mux/3
  From145/1 -> Mux24/2
  Demux9/5 -> Goto68/1  "pitch_d"
  From17/1 -> Mux4/1  "e"
  Demux8/5 -> Mux32/2  "e_pitch"
  Mux34/1 -> [angular_pose]
  [pose_x] -> Mux9/1
  Demux10/2 -> Goto51/1
  [pose_roll] -> Mux18/1
  [pose_z] -> Mux7/1
  Mux30/1 -> Mux34/2
  [des_y] -> Mux11/2
  Demux11/3 -> Mux36/3  "k_z"
  Demux7/6 -> [des_yaw]  "yaw_d"
  Mux4/1 -> To Workspace2/1
  From19/1 -> Mux6/2
  From134/1 -> Mux2/3
  Mux38/1 -> [angular_gain]
  Mux18/1 -> Mux34/1
  Demux11/5 -> Mux38/2  "k_pitch"
  Demux4/2 -> Goto42/1
  [Kt] -> Demux11/1  "k"
  Mux32/1 -> [angular_error]
  [qd] -> Demux7/1  "qd"
  Demux8/2 -> Mux31/2  "e_y"
  From143/1 -> Mux5/4
  From146/1 -> Mux26/2
  Mux27/1 -> pose vs pose_q/5
  [des_z] -> Mux7/2
  From147/1 -> Mux27/2
  From142/1 -> Mux5/3
  From140/1 -> Mux5/1
  From136/1 -> Mux3/2  "pose_dot"
  From107/1 -> Mux23/1
  Mux25/1 -> pose vs pose_q/6
  q/1 -> Bus Selector/1
  Bus Selector/1 -> [pos]  "<pos>"
  Bus Selector/2 -> [BF_att]  "<bf_att>"
  qd/1 -> Bus Selector1/1
  u/1 -> Bus Selector2/1
  Bus Selector2/1 -> Terminator/1  "<F_u>"
  Bus Selector2/2 -> Mux15/1  "<B-F_u>"
  Bus Selector2/3 -> Mux15/2  "<tau>"
  perb/1 -> Bus Selector3/1
  Bus Selector3/1 -> [drag_forces]  "<wind_perb>"
  [thrust] -> HEXA CAD ANSFT/3
  [forces] -> HEXA CAD ANSFT/6
  [torques] -> HEXA CAD ANSFT/9
  [drag_forces] -> HEXA CAD ANSFT/12  "drag forces"
  Bus Selector2/4 -> Mux14/1  "<sigma>"
  Demux/6 -> Mux10/3  "sig_yaw"
  Demux/5 -> Mux10/2  "sig_theta"
  Demux/3 -> Mux8/3  "sig_z"
  Demux/1 -> Mux8/1  "sig_x"
  Demux/4 -> Mux10/1  "sig_roll"
  Mux10/1 -> [sig_ang]
  Mux8/1 -> [sig_lin]
  [sigma] -> Demux/1
  Demux/2 -> Mux8/2  "sig_y"
  [sig_lin] -> HEXA CAD ANSFT/10
  [sig_ang] -> HEXA CAD ANSFT/11
  Demux2/2 -> [pose_pitch]  "pitch"
  Demux2/3 -> [pose_yaw]  "yaw"
  Demux2/1 -> [pose_roll]  "roll"
  Bus Selector2/8 -> [Kt]  "<Kt>"
  Bus Selector2/7 -> Mux13/2  "<eta_e>"
  Bus Selector2/6 -> Mux13/1  "<gamma_e>"
  Bus Selector2/5 -> Mux14/2  "<sigma_att>"
  Mux13/1 -> [error]
  Mux14/1 -> [sigma]
  Mux15/1 -> [F]
  Mux16/1 -> [qd]
  Bus Selector1/1 -> Mux16/1  "<xyz_d>"
  Bus Selector1/2 -> Quaternions to Rotation Angles/1  "<qd>"
  Quaternions to Rotation Angles/1 -> Mux16/2

== system Hexa_CAD_quaternion_ANSFT/6DoF_Dynamics/APC_8X3_8_Slow_Flyer_1_RIGID ==
  ReferenceFrame : sm_lib/Frames and Transforms/Reference Frame
  Solid : sm_lib/Body Elements/File Solid  ExtGeomFileName=APC 8X3.8 Slow Flyer_Valor predeterminado_sldprt.STEP  UnitType=FromFile  ExtGeomFileUnits=m  StepReaderType=HEX  ExportConvexHullGeometry=off  InertiaType=Custom  BasedOnType=DensityFromFile  Density=1000  DensityUnits=kg/m^3  Mass=smiData.Solid(8).mass  MassUnits=kg  CenterOfMass=smiData.Solid(8).CoM  CenterOfMassUnits=mm  MomentsOfInertia=smiData.Solid(8).MoI  MomentsOfInertiaUnits=kg*mm^2  ProductsOfInertia=smiData.Solid(8).PoI  ProductsOfInertiaUnits=kg*mm^2  GraphicType=FromGeometry  MarkerShape=Sphere  MarkerSize=10  GraphicVisPropType=SimpleVisualProperties  GraphicDiffuseColor=smiData.Solid(8).color  GraphicOpacity=smiData.Solid(8).opacity  GraphicSpecularColor=[0.5 0.5 0.5 1.0]  GraphicAmbientColor=[0.15 0.15 0.15 1.0]  GraphicEmissiveColor=[0.0 0.0 0.0 1.0]  GraphicShininess=75  DoExposeReferenceFrame=on  SerializedFrames=<Frames/>
  Transform : sm_lib/Frames and Transforms/Rigid Transform  RotationMethod=ArbitraryAxis  FollAlignAxisA=+X  BaseAlignAxisA=+Y  FollAlignAxisB=+Y  BaseAlignAxisB=+Z  RotationStandardAxis=+Z  RotationAngle=smiData.RigidTransform(20).angle  RotationAngleUnits=rad  RotationArbitraryAxis=smiData.RigidTransform(20).axis  RotationSequenceAxes=FollowerAxes  RotationSequence=XYX  RotationSequenceAngles=[0 0 0]  RotationSequenceAnglesUnits=deg  RotationMatrix=[1 0 0; 0 1 0; 0 0 1]  Quaternion=[1 0 0 0]  TranslationMethod=Cartesian  TranslationCartesianOffset=smiData.RigidTransform(20).translation  TranslationCartesianOffsetUnits=mm  TranslationStandardAxis=+Z  TranslationStandardOffset=0  TranslationStandardOffsetUnits=m  TranslationROffset=0  TranslationROffsetUnits=m  TranslationThetaOffset=0  TranslationThetaOffsetUnits=deg  TranslationZOffset=0  TranslationZOffsetUnits=m
  F : PMIOPort  Side=Left
  connections:
  ReferenceFrame/RConn1 -- Solid/RConn1 -- Transform/LConn1
  Transform/RConn1 -- F/RConn1

== system Hexa_CAD_quaternion_ANSFT/6DoF_Dynamics/APC_8X3_8_Slow_Flyer_2_RIGID ==
  ReferenceFrame : sm_lib/Frames and Transforms/Reference Frame
  Solid : sm_lib/Body Elements/File Solid  ExtGeomFileName=APC 8X3.8 Slow Flyer_Valor predeterminado_sldprt.STEP  UnitType=FromFile  ExtGeomFileUnits=m  StepReaderType=HEX  ExportConvexHullGeometry=off  InertiaType=Custom  BasedOnType=DensityFromFile  Density=1000  DensityUnits=kg/m^3  Mass=smiData.Solid(8).mass  MassUnits=kg  CenterOfMass=smiData.Solid(8).CoM  CenterOfMassUnits=mm  MomentsOfInertia=smiData.Solid(8).MoI  MomentsOfInertiaUnits=kg*mm^2  ProductsOfInertia=smiData.Solid(8).PoI  ProductsOfInertiaUnits=kg*mm^2  GraphicType=FromGeometry  MarkerShape=Sphere  MarkerSize=10  GraphicVisPropType=SimpleVisualProperties  GraphicDiffuseColor=smiData.Solid(8).color  GraphicOpacity=smiData.Solid(8).opacity  GraphicSpecularColor=[0.5 0.5 0.5 1.0]  GraphicAmbientColor=[0.15 0.15 0.15 1.0]  GraphicEmissiveColor=[0.0 0.0 0.0 1.0]  GraphicShininess=75  DoExposeReferenceFrame=on  SerializedFrames=<Frames/>
  Transform : sm_lib/Frames and Transforms/Rigid Transform  RotationMethod=ArbitraryAxis  FollAlignAxisA=+X  BaseAlignAxisA=+Y  FollAlignAxisB=+Y  BaseAlignAxisB=+Z  RotationStandardAxis=+Z  RotationAngle=smiData.RigidTransform(26).angle  RotationAngleUnits=rad  RotationArbitraryAxis=smiData.RigidTransform(26).axis  RotationSequenceAxes=FollowerAxes  RotationSequence=XYX  RotationSequenceAngles=[0 0 0]  RotationSequenceAnglesUnits=deg  RotationMatrix=[1 0 0; 0 1 0; 0 0 1]  Quaternion=[1 0 0 0]  TranslationMethod=Cartesian  TranslationCartesianOffset=smiData.RigidTransform(26).translation  TranslationCartesianOffsetUnits=mm  TranslationStandardAxis=+Z  TranslationStandardOffset=0  TranslationStandardOffsetUnits=m  TranslationROffset=0  TranslationROffsetUnits=m  TranslationThetaOffset=0  TranslationThetaOffsetUnits=deg  TranslationZOffset=0  TranslationZOffsetUnits=m
  F : PMIOPort  Side=Left
  connections:
  ReferenceFrame/RConn1 -- Solid/RConn1 -- Transform/LConn1
  Transform/RConn1 -- F/RConn1

== system Hexa_CAD_quaternion_ANSFT/6DoF_Dynamics/APC_8X3_8_Slow_Flyer_3_RIGID ==
  ReferenceFrame : sm_lib/Frames and Transforms/Reference Frame
  Solid : sm_lib/Body Elements/File Solid  ExtGeomFileName=APC 8X3.8 Slow Flyer_Valor predeterminado_sldprt.STEP  UnitType=FromFile  ExtGeomFileUnits=m  StepReaderType=HEX  ExportConvexHullGeometry=off  InertiaType=Custom  BasedOnType=DensityFromFile  Density=1000  DensityUnits=kg/m^3  Mass=smiData.Solid(8).mass  MassUnits=kg  CenterOfMass=smiData.Solid(8).CoM  CenterOfMassUnits=mm  MomentsOfInertia=smiData.Solid(8).MoI  MomentsOfInertiaUnits=kg*mm^2  ProductsOfInertia=smiData.Solid(8).PoI  ProductsOfInertiaUnits=kg*mm^2  GraphicType=FromGeometry  MarkerShape=Sphere  MarkerSize=10  GraphicVisPropType=SimpleVisualProperties  GraphicDiffuseColor=smiData.Solid(8).color  GraphicOpacity=smiData.Solid(8).opacity  GraphicSpecularColor=[0.5 0.5 0.5 1.0]  GraphicAmbientColor=[0.15 0.15 0.15 1.0]  GraphicEmissiveColor=[0.0 0.0 0.0 1.0]  GraphicShininess=75  DoExposeReferenceFrame=on  SerializedFrames=<Frames/>
  Transform : sm_lib/Frames and Transforms/Rigid Transform  RotationMethod=ArbitraryAxis  FollAlignAxisA=+X  BaseAlignAxisA=+Y  FollAlignAxisB=+Y  BaseAlignAxisB=+Z  RotationStandardAxis=+Z  RotationAngle=smiData.RigidTransform(28).angle  RotationAngleUnits=rad  RotationArbitraryAxis=smiData.RigidTransform(28).axis  RotationSequenceAxes=FollowerAxes  RotationSequence=XYX  RotationSequenceAngles=[0 0 0]  RotationSequenceAnglesUnits=deg  RotationMatrix=[1 0 0; 0 1 0; 0 0 1]  Quaternion=[1 0 0 0]  TranslationMethod=Cartesian  TranslationCartesianOffset=smiData.RigidTransform(28).translation  TranslationCartesianOffsetUnits=mm  TranslationStandardAxis=+Z  TranslationStandardOffset=0  TranslationStandardOffsetUnits=m  TranslationROffset=0  TranslationROffsetUnits=m  TranslationThetaOffset=0  TranslationThetaOffsetUnits=deg  TranslationZOffset=0  TranslationZOffsetUnits=m
  F : PMIOPort  Side=Left
  connections:
  ReferenceFrame/RConn1 -- Solid/RConn1 -- Transform/LConn1
  Transform/RConn1 -- F/RConn1

== system Hexa_CAD_quaternion_ANSFT/6DoF_Dynamics/APC_8X3_8_Slow_Flyer_4_RIGID ==
  ReferenceFrame : sm_lib/Frames and Transforms/Reference Frame
  Solid : sm_lib/Body Elements/File Solid  ExtGeomFileName=APC 8X3.8 Slow Flyer_Valor predeterminado_sldprt.STEP  UnitType=FromFile  ExtGeomFileUnits=m  StepReaderType=HEX  ExportConvexHullGeometry=off  InertiaType=Custom  BasedOnType=DensityFromFile  Density=1000  DensityUnits=kg/m^3  Mass=smiData.Solid(8).mass  MassUnits=kg  CenterOfMass=smiData.Solid(8).CoM  CenterOfMassUnits=mm  MomentsOfInertia=smiData.Solid(8).MoI  MomentsOfInertiaUnits=kg*mm^2  ProductsOfInertia=smiData.Solid(8).PoI  ProductsOfInertiaUnits=kg*mm^2  GraphicType=FromGeometry  MarkerShape=Sphere  MarkerSize=10  GraphicVisPropType=SimpleVisualProperties  GraphicDiffuseColor=smiData.Solid(8).color  GraphicOpacity=smiData.Solid(8).opacity  GraphicSpecularColor=[0.5 0.5 0.5 1.0]  GraphicAmbientColor=[0.15 0.15 0.15 1.0]  GraphicEmissiveColor=[0.0 0.0 0.0 1.0]  GraphicShininess=75  DoExposeReferenceFrame=on  SerializedFrames=<Frames/>
  Transform : sm_lib/Frames and Transforms/Rigid Transform  RotationMethod=ArbitraryAxis  FollAlignAxisA=+X  BaseAlignAxisA=+Y  FollAlignAxisB=+Y  BaseAlignAxisB=+Z  RotationStandardAxis=+Z  RotationAngle=smiData.RigidTransform(34).angle  RotationAngleUnits=rad  RotationArbitraryAxis=smiData.RigidTransform(34).axis  RotationSequenceAxes=FollowerAxes  RotationSequence=XYX  RotationSequenceAngles=[0 0 0]  RotationSequenceAnglesUnits=deg  RotationMatrix=[1 0 0; 0 1 0; 0 0 1]  Quaternion=[1 0 0 0]  TranslationMethod=Cartesian  TranslationCartesianOffset=smiData.RigidTransform(34).translation  TranslationCartesianOffsetUnits=mm  TranslationStandardAxis=+Z  TranslationStandardOffset=0  TranslationStandardOffsetUnits=m  TranslationROffset=0  TranslationROffsetUnits=m  TranslationThetaOffset=0  TranslationThetaOffsetUnits=deg  TranslationZOffset=0  TranslationZOffsetUnits=m
  F : PMIOPort  Side=Left
  connections:
  ReferenceFrame/RConn1 -- Solid/RConn1 -- Transform/LConn1
  Transform/RConn1 -- F/RConn1

== system Hexa_CAD_quaternion_ANSFT/6DoF_Dynamics/APC_8X3_8_Slow_Flyer_5_RIGID ==
  ReferenceFrame : sm_lib/Frames and Transforms/Reference Frame
  Solid : sm_lib/Body Elements/File Solid  ExtGeomFileName=APC 8X3.8 Slow Flyer_Valor predeterminado_sldprt.STEP  UnitType=FromFile  ExtGeomFileUnits=m  StepReaderType=HEX  ExportConvexHullGeometry=off  InertiaType=Custom  BasedOnType=DensityFromFile  Density=1000  DensityUnits=kg/m^3  Mass=smiData.Solid(8).mass  MassUnits=kg  CenterOfMass=smiData.Solid(8).CoM  CenterOfMassUnits=mm  MomentsOfInertia=smiData.Solid(8).MoI  MomentsOfInertiaUnits=kg*mm^2  ProductsOfInertia=smiData.Solid(8).PoI  ProductsOfInertiaUnits=kg*mm^2  GraphicType=FromGeometry  MarkerShape=Sphere  MarkerSize=10  GraphicVisPropType=SimpleVisualProperties  GraphicDiffuseColor=smiData.Solid(8).color  GraphicOpacity=smiData.Solid(8).opacity  GraphicSpecularColor=[0.5 0.5 0.5 1.0]  GraphicAmbientColor=[0.15 0.15 0.15 1.0]  GraphicEmissiveColor=[0.0 0.0 0.0 1.0]  GraphicShininess=75  DoExposeReferenceFrame=on  SerializedFrames=<Frames/>
  Transform : sm_lib/Frames and Transforms/Rigid Transform  RotationMethod=ArbitraryAxis  FollAlignAxisA=+X  BaseAlignAxisA=+Y  FollAlignAxisB=+Y  BaseAlignAxisB=+Z  RotationStandardAxis=+Z  RotationAngle=smiData.RigidTransform(36).angle  RotationAngleUnits=rad  RotationArbitraryAxis=smiData.RigidTransform(36).axis  RotationSequenceAxes=FollowerAxes  RotationSequence=XYX  RotationSequenceAngles=[0 0 0]  RotationSequenceAnglesUnits=deg  RotationMatrix=[1 0 0; 0 1 0; 0 0 1]  Quaternion=[1 0 0 0]  TranslationMethod=Cartesian  TranslationCartesianOffset=smiData.RigidTransform(36).translation  TranslationCartesianOffsetUnits=mm  TranslationStandardAxis=+Z  TranslationStandardOffset=0  TranslationStandardOffsetUnits=m  TranslationROffset=0  TranslationROffsetUnits=m  TranslationThetaOffset=0  TranslationThetaOffsetUnits=deg  TranslationZOffset=0  TranslationZOffsetUnits=m
  F : PMIOPort  Side=Left
  connections:
  ReferenceFrame/RConn1 -- Solid/RConn1 -- Transform/LConn1
  Transform/RConn1 -- F/RConn1

== system Hexa_CAD_quaternion_ANSFT/6DoF_Dynamics/APC_8X3_8_Slow_Flyer_6_RIGID ==
  ReferenceFrame : sm_lib/Frames and Transforms/Reference Frame
  Solid : sm_lib/Body Elements/File Solid  ExtGeomFileName=APC 8X3.8 Slow Flyer_Valor predeterminado_sldprt.STEP  UnitType=FromFile  ExtGeomFileUnits=m  StepReaderType=HEX  ExportConvexHullGeometry=off  InertiaType=Custom  BasedOnType=DensityFromFile  Density=1000  DensityUnits=kg/m^3  Mass=smiData.Solid(8).mass  MassUnits=kg  CenterOfMass=smiData.Solid(8).CoM  CenterOfMassUnits=mm  MomentsOfInertia=smiData.Solid(8).MoI  MomentsOfInertiaUnits=kg*mm^2  ProductsOfInertia=smiData.Solid(8).PoI  ProductsOfInertiaUnits=kg*mm^2  GraphicType=FromGeometry  MarkerShape=Sphere  MarkerSize=10  GraphicVisPropType=SimpleVisualProperties  GraphicDiffuseColor=smiData.Solid(8).color  GraphicOpacity=smiData.Solid(8).opacity  GraphicSpecularColor=[0.5 0.5 0.5 1.0]  GraphicAmbientColor=[0.15 0.15 0.15 1.0]  GraphicEmissiveColor=[0.0 0.0 0.0 1.0]  GraphicShininess=75  DoExposeReferenceFrame=on  SerializedFrames=<Frames/>
  Transform : sm_lib/Frames and Transforms/Rigid Transform  RotationMethod=ArbitraryAxis  FollAlignAxisA=+X  BaseAlignAxisA=+Y  FollAlignAxisB=+Y  BaseAlignAxisB=+Z  RotationStandardAxis=+Z  RotationAngle=smiData.RigidTransform(42).angle  RotationAngleUnits=rad  RotationArbitraryAxis=smiData.RigidTransform(42).axis  RotationSequenceAxes=FollowerAxes  RotationSequence=XYX  RotationSequenceAngles=[0 0 0]  RotationSequenceAnglesUnits=deg  RotationMatrix=[1 0 0; 0 1 0; 0 0 1]  Quaternion=[1 0 0 0]  TranslationMethod=Cartesian  TranslationCartesianOffset=smiData.RigidTransform(42).translation  TranslationCartesianOffsetUnits=mm  TranslationStandardAxis=+Z  TranslationStandardOffset=0  TranslationStandardOffsetUnits=m  TranslationROffset=0  TranslationROffsetUnits=m  TranslationThetaOffset=0  TranslationThetaOffsetUnits=deg  TranslationZOffset=0  TranslationZOffsetUnits=m
  F : PMIOPort  Side=Left
  connections:
  ReferenceFrame/RConn1 -- Solid/RConn1 -- Transform/LConn1
  Transform/RConn1 -- F/RConn1
